simulink model "Backstepping_Quadrator_Position"  (R2018a)
settings: Solver=ode4  StartTime=0.0  StopTime=20  FixedStep=1e-4  MaxStep=1e-3  MinStep=1e-4  RelTol=1e-3
libraries: simulink x13
settings Model: Creator=oussa  LastModifiedBy=oussa

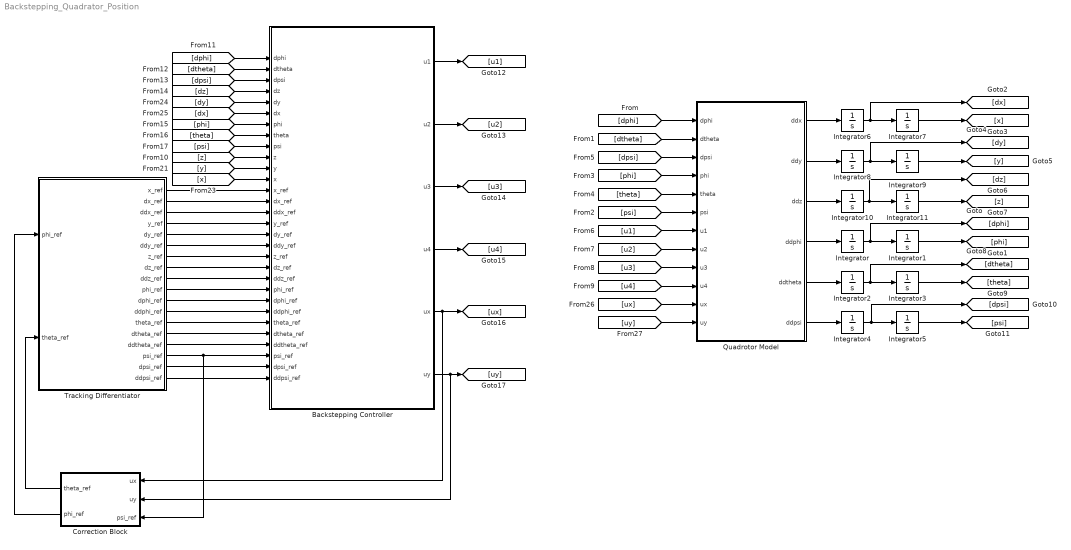
== system Backstepping_Quadrator_Position ==
  Backstepping Controller : MATLAB Function  TreatAsAtomicUnit=on
  Correction Block : Subsystem
  Integrator : Integrator  InitialCondition=0.3
  Integrator{1..11} (11 alike) : Integrator
  Quadrotor Model : MATLAB Function  TreatAsAtomicUnit=on
  Tracking Differentiator : Subsystem
  wires:
  Quadrotor Model/4(ddphi) -> Integrator/1
  Quadrotor Model/5(ddtheta) -> Integrator2/1
  Quadrotor Model/6(ddpsi) -> Integrator4/1
  Integrator10/1 -> [dz], Integrator11/1
  Integrator8/1 -> [dy], Integrator9/1
  Quadrotor Model/1(ddx) -> Integrator6/1
  Quadrotor Model/3(ddz) -> Integrator10/1
  Quadrotor Model/2(ddy) -> Integrator8/1
  Integrator4/1 -> [dpsi], Integrator5/1
  Integrator2/1 -> Integrator3/1, [dtheta]
  Integrator/1 -> Integrator1/1, [dphi]
  Integrator1/1 -> [phi]
  Integrator7/1 -> [x]
  Integrator6/1 -> [dx], Integrator7/1
  Integrator9/1 -> [y]
  Integrator11/1 -> [z]
  Integrator3/1 -> [theta]
  Integrator5/1 -> [psi]
  [dphi] -> Quadrotor Model/1(dphi)
  [dtheta] -> Quadrotor Model/2(dtheta)
  [phi] -> Quadrotor Model/4(phi)
  [theta] -> Quadrotor Model/5(theta)
  [dpsi] -> Quadrotor Model/3(dpsi)
  [psi] -> Quadrotor Model/6(psi)
  [u1] -> Quadrotor Model/7(u1)
  [u2] -> Quadrotor Model/8(u2)
  [u3] -> Quadrotor Model/9(u3)
  [u4] -> Quadrotor Model/10(u4)
  Backstepping Controller/2(u2) -> [u2]
  [dphi] -> Backstepping Controller/1(dphi)
  [dtheta] -> Backstepping Controller/2(dtheta)
  [dpsi] -> Backstepping Controller/3(dpsi)
  [z] -> Backstepping Controller/10(z)
  [y] -> Backstepping Controller/11(y)
  [x] -> Backstepping Controller/12(x)
  [psi] -> Backstepping Controller/9(psi)
  [theta] -> Backstepping Controller/8(theta)
  [phi] -> Backstepping Controller/7(phi)
  [dz] -> Backstepping Controller/4(dz)
  [dy] -> Backstepping Controller/5(dy)
  [dx] -> Backstepping Controller/6(dx)
  Backstepping Controller/1(u1) -> [u1]
  Backstepping Controller/3(u3) -> [u3]
  Backstepping Controller/4(u4) -> [u4]
  Tracking Differentiator/1("x_ref ") -> Backstepping Controller/13(x_ref)
  Tracking Differentiator/2(dx_ref) -> Backstepping Controller/14(dx_ref)
  Tracking Differentiator/3(ddx_ref) -> Backstepping Controller/15(ddx_ref)
  Tracking Differentiator/4("y_ref ") -> Backstepping Controller/16(y_ref)
  Tracking Differentiator/5(dy_ref) -> Backstepping Controller/17(dy_ref)
  Tracking Differentiator/6(ddy_ref) -> Backstepping Controller/18(ddy_ref)
  Tracking Differentiator/7("z_ref ") -> Backstepping Controller/19(z_ref)
  Tracking Differentiator/8(dz_ref) -> Backstepping Controller/20(dz_ref)
  Tracking Differentiator/9(ddz_ref) -> Backstepping Controller/21(ddz_ref)
  Tracking Differentiator/10("phi_ref ") -> Backstepping Controller/22(phi_ref)
  Tracking Differentiator/11(dphi_ref) -> Backstepping Controller/23(dphi_ref)
  Tracking Differentiator/12(ddphi_ref) -> Backstepping Controller/24(ddphi_ref)
  Tracking Differentiator/13("theta_ref ") -> Backstepping Controller/25(theta_ref)
  Tracking Differentiator/14("dtheta_ref ") -> Backstepping Controller/26(dtheta_ref)
  Tracking Differentiator/15(ddtheta_ref) -> Backstepping Controller/27(ddtheta_ref)
  Tracking Differentiator/17(dpsi_ref) -> Backstepping Controller/29(dpsi_ref)
  Tracking Differentiator/18(ddpsi_ref) -> Backstepping Controller/30(ddpsi_ref)
  Backstepping Controller/6(uy) -> Correction Block/2(uy), [uy]
  Tracking Differentiator/16("psi_ref ") -> Correction Block/3(psi_ref), Backstepping Controller/28(psi_ref)
  [uy] -> Quadrotor Model/12(uy)
  [ux] -> Quadrotor Model/11(ux)
  Backstepping Controller/5(ux) -> [ux], Correction Block/1(ux)
  Correction Block/1(theta_ref) -> Tracking Differentiator/2(theta_ref)
  Correction Block/2(phi_ref) -> Tracking Differentiator/1(phi_ref)

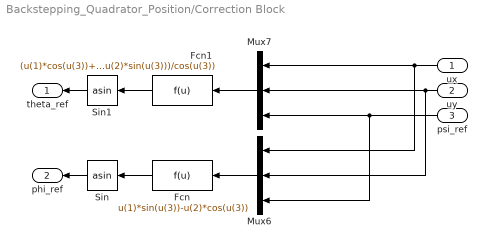
== system Backstepping_Quadrator_Position/Correction Block ==
  ux : Inport
  uy : Inport  Port=2
  psi_ref : Inport  Port=3
  Fcn : Fcn  Expr=u(1)*sin(u(3))-u(2)*cos(u(3))
  Fcn1 : Fcn  Expr=(u(1)*cos(u(3))+u(2)*sin(u(3)))/cos(u(3))
  Mux6 : Mux  Inputs=3
  Mux7 : Mux  Inputs=3
  Sin : Trigonometry  Operator=asin
  Sin1 : Trigonometry  Operator=asin  OutputSignalType=real
  theta_ref : Outport
  phi_ref : Outport  Port=2
  wires:
  Fcn1/1 -> Sin1/1
  ux/1 -> Mux7/1, Mux6/1
  psi_ref/1 -> Mux6/3, Mux7/3
  Mux7/1 -> Fcn1/1
  uy/1 -> Mux7/2, Mux6/2
  Mux6/1 -> Fcn/1
  Fcn/1 -> Sin/1
  Sin1/1 -> theta_ref/1
  Sin/1 -> phi_ref/1

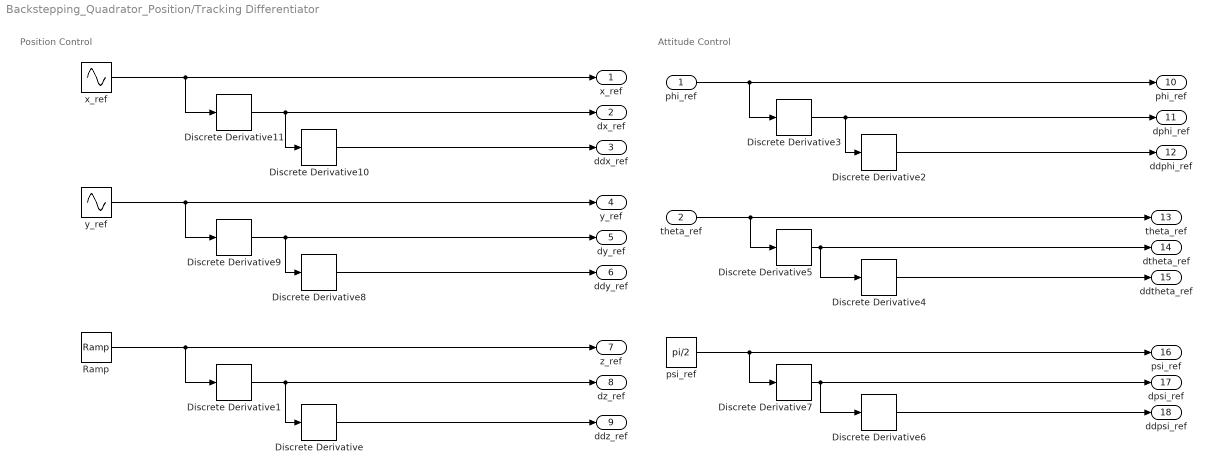
== system Backstepping_Quadrator_Position/Tracking Differentiator ==
  note: Attitude Control
  note: Position Control
  phi_ref : Inport
  theta_ref : Inport  Port=2
  Discrete Derivative{,1..11} (12 alike) : simulink/Discrete/Discrete Derivative  gainval=eps  ICPrevScaledInput=0.0  OutMin=[]  OutMax=[]  OutDataType=fixdt(1, 16)  OutScaling=2^-10  DoSatur=off
  Ramp : simulink/Sources/Ramp  slope=0.1  start=0  InitialOutput=0
  psi_ref : Constant  Value=pi/2
  x_ref : Sin  Frequency=2*pi*0.5  Phase=pi/2  SampleTime=0
  y_ref : Sin  Frequency=2*pi*0.5  SampleTime=0
  "x_ref " : Outport
  dx_ref : Outport  Port=2
  ddx_ref : Outport  Port=3
  "y_ref " : Outport  Port=4
  dy_ref : Outport  Port=5
  ddy_ref : Outport  Port=6
  "z_ref " : Outport  Port=7
  dz_ref : Outport  Port=8
  ddz_ref : Outport  Port=9
  "phi_ref " : Outport  Port=10
  dphi_ref : Outport  Port=11
  ddphi_ref : Outport  Port=12
  "theta_ref " : Outport  Port=13
  "dtheta_ref " : Outport  Port=14
  ddtheta_ref : Outport  Port=15
  "psi_ref " : Outport  Port=16
  dpsi_ref : Outport  Port=17
  ddpsi_ref : Outport  Port=18
  wires:
  Discrete Derivative/1 -> ddz_ref/1
  Discrete Derivative4/1 -> ddtheta_ref/1
  Discrete Derivative1/1 -> Discrete Derivative/1, dz_ref/1
  Discrete Derivative3/1 -> dphi_ref/1, Discrete Derivative2/1
  Discrete Derivative5/1 -> "dtheta_ref "/1, Discrete Derivative4/1
  Ramp/1 -> "z_ref "/1, Discrete Derivative1/1
  phi_ref/1 -> "phi_ref "/1, Discrete Derivative3/1
  Discrete Derivative8/1 -> ddy_ref/1
  Discrete Derivative9/1 -> Discrete Derivative8/1, dy_ref/1
  x_ref/1 -> "x_ref "/1, Discrete Derivative11/1
  Discrete Derivative11/1 -> Discrete Derivative10/1, dx_ref/1
  Discrete Derivative10/1 -> ddx_ref/1
  Discrete Derivative2/1 -> ddphi_ref/1
  theta_ref/1 -> Discrete Derivative5/1, "theta_ref "/1
  psi_ref/1 -> Discrete Derivative7/1, "psi_ref "/1
  Discrete Derivative7/1 -> dpsi_ref/1, Discrete Derivative6/1
  Discrete Derivative6/1 -> ddpsi_ref/1
  y_ref/1 -> "y_ref "/1, Discrete Derivative9/1

== matlab function Backstepping_Quadrator_Position/Backstepping Controller ==
  data: dphi input; dtheta input; dpsi input; dz input; dy input; dx input; phi input; theta input; psi input; z input; y input; x input; x_ref input; dx_ref input; ddx_ref input; y_ref input; dy_ref input; ddy_ref input; z_ref input; dz_ref input; ddz_ref input; phi_ref input; dphi_ref input; ddphi_ref input; theta_ref input; dtheta_ref input; u1 output; u2 output; u3 output; u4 output; ddtheta_ref input; psi_ref input; dpsi_ref input; ddpsi_ref input; ux output; uy output
function [u1,u2,u3,u4,ux,uy] = Backstepping_Controller(dphi,dtheta,dpsi,dz,dy,dx,phi,theta,psi,z,y,x,x_ref,dx_ref,ddx_ref,y_ref,dy_ref,ddy_ref,z_ref,dz_ref,ddz_ref,phi_ref,dphi_ref,ddphi_ref,theta_ref,dtheta_ref,ddtheta_ref,psi_ref,dpsi_ref,ddpsi_ref)
m = 2;
Ix = 1.25;
Iy = 1.25;
Iz = 2.2;
Ir = 1;
g = 9.8;
w = 100;

a1 = (Iy-Iz)/Ix; a2 = -Ir/Ix*w; b1 = 1/Ix;
a3 = (Iz-Ix)/Iy; a4 = Ir/Iy*w; b2 = 1/Iy;
a5= (Ix-Iy)/Iz; b3 = 1/Iz;

k1 = 100;
k2 = k1;
k3 = k1;
k4 = k1;
k5 = k1;
k6 = k1;
k7 = k1;
k8 = k1;
k9 = k1;
k10 = k1;
k11 = k1;
k12 = k1;


e1 = phi_ref-phi;
e2 = dphi-k1*e1-dphi_ref;
u2 = 1/b1*(-k2*e2+e1+ddphi_ref-k1*(e2+k1*e1)-a1*dtheta*dpsi-a2*dtheta*w);

e3 = theta_ref-theta;
e4 = dtheta-dtheta_ref-k3*e3;
u3 = 1/b2*(-k4*e4+e3-a3*dphi*dpsi-a4*w*dphi+ddtheta_ref-k3*(e4+k3*e3));

e5 = psi_ref-psi;
e6 = dpsi-dpsi_ref-k5*e5;
u4 = 1/b3*(-k6*e6+e5-a5*dphi*dtheta+ddpsi_ref-k5*(e6+k5*e5));

e7 = z_ref-z;
e8 = dz-dz_ref-k7*e7;
u1 = m/(cos(phi)*cos(theta))*(-k8*e8+e7+g-k7*(e8+k7*e7)+ddz_ref);

e9 = y_ref-y;
e10 = dy-dy_ref-k9*e9;
uy = m/u1*(e9-k10*e10-k9*(k9*e9+e10)+ddy_ref);

e11 = x_ref-x;
e12 = dx-k11*e11-dx_ref;
ux = m/u1*(e11-k12*e12-k11*(k11*e11+e12)+ddx_ref);
end

== matlab function Backstepping_Quadrator_Position/Quadrotor Model ==
  data: ddx output size=1; dphi input size=1; dtheta input size=1; dpsi input size=1; phi input size=1; theta input size=1; psi input size=1; u1 input size=1; u2 input size=1; u3 input size=1; u4 input size=1; ddy output size=1; ddz output size=1; ddphi output size=1; ddtheta output size=1; ddpsi output size=1; ux input; uy input
function [ddx,ddy,ddz,ddphi,ddtheta,ddpsi] = Quadrotor(dphi,dtheta,dpsi,phi,theta,psi,u1,u2,u3,u4,ux,uy)
m = 2;
Ix = 1.25;
Iy = 1.25;
Iz = 2.2;
Ir = 1;
g = 9.8;
w = 1;
a1 = (Iy-Iz)/Ix; a2 = -Ir/Ix*w; a3 = 1/Ix;
b1 = (Iz-Ix)/Iy; b2 = Ir/Iy*w; b3 = 1/Iy;
c1= (Ix-Iy)/Iz; c2 = 1/Iz;

ddx = ux*u1/m;
ddy = uy*u1/m;
ddz = -g+(cos(theta)*cos(phi))*u1/m;


ddphi = a1*dtheta*dpsi+a2*w*dtheta+a3*u2;
ddtheta = b1*dpsi*dphi+b2*dphi+b3*u3;
ddpsi = c1*dtheta*dphi+c2*u4;

end
